simulink model "EcoSIM3_P2_C2_WIP"  (R2014b)
settings: Solver=ode1  SolverMode=SingleTasking  StartTime=0.0  StopTime=4  FixedStep=0.01  RelTol=1e-3
PostLoadFcn:
  | %, if any(exist('dsrtsu_mdlpostloadfcn', 'file') == [2, 3, 6]), try dsrtsu_mdlpostloadfcn('Execute', bdroot); catch fprintf('Error in PostLoadFcn (dsrtsu_mdlpostloadfcn) for model "%s":\n %s\n', bdroot, lasterr); end, end,
InitFcn:
  | tic
  | %Startup_EcoSIM
undefined symbols (not defined in the file or in its folder): canChannel, Controls, DriveCycles, Driver, EM_EFF_MAP, EM_PwrLoss_MAP, EngPwr, EngSpd, EngTrq, Glbl, Overwritten_Mode, Plants, Power, sigbuilder_block, Torque, Trialmap, Veh_Dynamics
libraries: simulink x135, canmsglib x113, fl_lib x104, canlib x89, nesl_utility x56, sdl_lib x29, dspsigops x6, dspswit3 x5, dspstat3 x2, commnoisgen2 x1, dspfdesign x1
(part 11 of 21)

== system EcoSIM3_P2_C2_WIP/Powertrain/Soft_ECUs_IO/From_Goto/Subsystem1/Engine_Relay ==
  In1 : Inport
  Constant4 : Constant
  Constant5 : Constant  Value=0
  Relay2 : Switch  Criteria=u2 > Threshold  Threshold=0.5
  Out1 : Outport
  wires:
  Relay2/1 -> Out1/1  "ICE_Powerup"
  Constant5/1 -> Relay2/3
  Constant4/1 -> Relay2/1
  In1/1 -> Relay2/2

== system EcoSIM3_P2_C2_WIP/Powertrain/Soft_ECUs_IO/VNT Kvaser/CANRx/BAS Receive ==
  Bus Creator12 : BusCreator  Inputs=1
  Bus Creator2 : BusCreator  Inputs=2
  CAN Receive : canlib/CAN Receive  BlockHandle=2745.0026  DeviceMenu=Kvaser Virtual 1 (Channel 1)  Device=Kvaser Virtual 1 (Channel 1)  ObjConstructor=canChannel('Kvaser', 'Virtual 1', 1)  EnableStandardIDsFilter=off  StandardIDs=102  EnableExtendedIDsFilter=off  ExtendedIDs=0  SampleTime=0.01  MsgsPerTimestep=1  StdIDsCombo=Allow only  ExtIDsCombo=Block all  InternalFilterUpdateStatus=on
  CAN Unpack : canmsglib/CAN Unpack  CANdbFile=C:\Users\EcoCAR_HIL\Documents\Khanna\EcoSIM3_P1_0_PHEV_TCU\Final_DBC\Engine_Transmission_BAS.dbc  MsgList=ECO_BAS_Receive_MSG102  MsgName=ECO_BAS_Receive_MSG102  MsgIDType=Standard (11-bit identifier)  MsgIdentifier=102  MsgLength=2  SignalInfo=BAS_Mode_Request$8$1$2$2$1$0$1$0$0$1$#BAS_Torque_Request_Nm$9$15$2$1$1$0$1.000000e-02$0$-1.638400e+02$1.638300e+02$#  NSignals=2  IDPort=off  TimestampPort=off  ErrorPort=off  RemotePort=off  LengthPort=off  StatusPort=off  StartBits=str2num('[int32(8);int32(9)]')  SignalSizes=str2num('[int32(1);int32(15)]')  ByteOrders=str2num('[int32(2);int32(2)]')  DataTypes=str2num('[int32(2);int32(1)]')  MultiplexTypes=str2num('[int32(1);int32(1)]')  MultiplexValues=str2num('[double(0);double(0)]')  Factors=str2num('[double(1);double(1.000000e-02)]')  Offsets=str2num('[double(0);double(0)]')  Minimums=str2num('[double(0);double(-1.638400e+02)]')  Maximums=str2num('[double(1);double(1.638300e+02)]')
      settings: DataFormat=CANdb specified signals
  Terminator6 : Terminator
  BAS_CAN : Outport
  wires:
  Bus Creator12/1 -> BAS_CAN/1  "BAS_CAN"
  Bus Creator2/1 -> Bus Creator12/1  "SetValues"
  CAN Receive/1 -> Terminator6/1
  CAN Unpack/1 -> Bus Creator2/1  "BAS_Mode_Request"
  CAN Unpack/2 -> Bus Creator2/2  "BAS_Torque_Request_Nm"
  CAN Receive/2 -> CAN Unpack/1

== system EcoSIM3_P2_C2_WIP/Powertrain/Soft_ECUs_IO/VNT Kvaser/CANRx/Brusa Receive ==
  Bus Creator4 : BusCreator  Inputs=2
  Ground : Ground
  Ground1 : Ground
  Brusa CAN : Outport
  wires:
  Bus Creator4/1 -> Brusa CAN/1  "Brusa_CAN"
  Ground/1 -> Bus Creator4/1  "Dummy1"
  Ground1/1 -> Bus Creator4/2  "Dummy2"

== system EcoSIM3_P2_C2_WIP/Powertrain/Soft_ECUs_IO/VNT Kvaser/CANRx/EM Receive ==
  Bus Creator : BusCreator  Inputs=1
  Bus Creator1 : BusCreator  Inputs=3
  CAN Receive1 : canlib/CAN Receive  BlockHandle=2767.0024  DeviceMenu=Kvaser Virtual 1 (Channel 2)  Device=Kvaser Virtual 1 (Channel 2)  ObjConstructor=canChannel('Kvaser', 'Virtual 1', 2)  EnableStandardIDsFilter=off  StandardIDs=192  EnableExtendedIDsFilter=off  ExtendedIDs=0  SampleTime=0.01  MsgsPerTimestep=1  StdIDsCombo=Allow only  ExtIDsCombo=Block all  InternalFilterUpdateStatus=on
  CAN Unpack2 : canmsglib/CAN Unpack  CANdbFile=C:\Users\EcoCAR_HIL\Documents\Khanna\EcoSIM3_P1_0_PHEV_TCU\Final_DBC\20150828 RMS PM CAN DB.dbc  MsgList=M192_Command_Message  MsgName=M192_Command_Message  MsgIDType=Standard (11-bit identifier)  MsgIdentifier=192  MsgLength=8  SignalInfo=Direction_Command$42$1$1$2$1$0$1$0$0$1$#Inverter_Discharge$41$1$1$2$1$0$1$0$0$1$#Inverter_Enable$40$1$1$2$1$0$1$0$0$1$#Speed_Command$16$16$1$1$1$0$1$0$-32768$32767$#Torque_Command$0$16$1$1$1$0$1.000000e-01$0$-3.276800e+03$3.276700e+03$#Torque_Limit_Command$48$16$1$1$1$0$1$0$-3.276800e+03$3.276700e+03$#  NSignals=6  IDPort=off  TimestampPort=off  ErrorPort=off  RemotePort=off  LengthPort=off  StatusPort=off  StartBits=str2num('[int32(42);int32(41);int32(40);int32(16);int32(0);int32(48)]')  SignalSizes=str2num('[int32(1);int32(1);int32(1);int32(16);int32(16);int32(16)]')  ByteOrders=str2num('[int32(1);int32(1);int32(1);int32(1);int32(1);int32(1)]')  DataTypes=str2num('[int32(2);int32(2);int32(2);int32(1);int32(1);int32(1)]')  MultiplexTypes=str2num('[int32(1);int32(1);int32(1);int32(1);int32(1);int32(1)]')  MultiplexValues=str2num('[double(0);double(0);double(0);double(0);double(0);double(0)]')  Factors=str2num('[double(1);double(1);double(1);double(1);double(1.000000e-01);double(1)]')  Offsets=str2num('[double(0);double(0);double(0);double(0);double(0);double(0)]')  Minimums=str2num('[double(0);double(0);double(0);double(-32768);double(-3.276800e+03);double(-3.276800e+03)]')  Maximums=str2num('[double(1);double(1);double(1);double(32767);double(3.276700e+03);double(3.276700e+03)]')
      settings: DataFormat=CANdb specified signals
  Terminator{5,7..9} (4 alike) : Terminator
  EM CAN : Outport
  wires:
  Bus Creator/1 -> EM CAN/1  "EM_CAN"
  Bus Creator1/1 -> Bus Creator/1  "M192_Command_Message"
  CAN Receive1/2 -> CAN Unpack2/1
  CAN Receive1/1 -> Terminator5/1
  CAN Unpack2/1 -> Bus Creator1/1  "Rotation_Direction"
  CAN Unpack2/3 -> Bus Creator1/2  "Inverter_Enable"
  CAN Unpack2/5 -> Bus Creator1/3  "Torque_Command"
  CAN Unpack2/2 -> Terminator7/1
  CAN Unpack2/4 -> Terminator8/1
  CAN Unpack2/6 -> Terminator9/1

== system EcoSIM3_P2_C2_WIP/Powertrain/Soft_ECUs_IO/VNT Kvaser/CANRx/ESS Receive ==
  Bus Creator5 : BusCreator
  Bus Creator6 : BusCreator  Inputs=1
  CAN Receive4 : canlib/CAN Receive  BlockHandle=2787.0027  DeviceMenu=Kvaser Virtual 1 (Channel 1)  Device=Kvaser Virtual 1 (Channel 1)  ObjConstructor=canChannel('Kvaser', 'Virtual 1', 1)  EnableStandardIDsFilter=off  StandardIDs=1024  EnableExtendedIDsFilter=off  ExtendedIDs=0  SampleTime=0.01  MsgsPerTimestep=1  StdIDsCombo=Allow only  ExtIDsCombo=Block all  InternalFilterUpdateStatus=on
  CAN Unpack4 : canmsglib/CAN Unpack  CANdbFile=C:\Users\EcoCAR_HIL\Documents\Khanna\EcoSIM3_P1_0_PHEV_TCU\Final_DBC\BCM_VehBus_Std.dbc  MsgList=BCM_Request  MsgName=BCM_Request  MsgIDType=Standard (11-bit identifier)  MsgIdentifier=1024  MsgLength=4  SignalInfo=hsc_bcm_enable$0$1$2$2$1$0$1$0$0$1$#hsc_bcm_epo$1$1$2$2$1$0$1$0$0$1$#hsc_bcm_leakage_ena$3$1$2$2$1$0$1$0$0$1$#hsc_bcm_mainc_close$2$1$2$2$1$0$1$0$0$1$#  NSignals=4  IDPort=off  TimestampPort=off  ErrorPort=off  RemotePort=off  LengthPort=off  StatusPort=off  StartBits=str2num('[int32(0);int32(1);int32(3);int32(2)]')  SignalSizes=str2num('[int32(1);int32(1);int32(1);int32(1)]')  ByteOrders=str2num('[int32(2);int32(2);int32(2);int32(2)]')  DataTypes=str2num('[int32(2);int32(2);int32(2);int32(2)]')  MultiplexTypes=str2num('[int32(1);int32(1);int32(1);int32(1)]')  MultiplexValues=str2num('[double(0);double(0);double(0);double(0)]')  Factors=str2num('[double(1);double(1);double(1);double(1)]')  Offsets=str2num('[double(0);double(0);double(0);double(0)]')  Minimums=str2num('[double(0);double(0);double(0);double(0)]')  Maximums=str2num('[double(1);double(1);double(1);double(1)]')
      settings: DataFormat=CANdb specified signals
  Terminator3 : Terminator
  ESS CAN : Outport
  wires:
  Bus Creator5/1 -> Bus Creator6/1  "BCM_Request"
  Bus Creator6/1 -> ESS CAN/1  "BCM_CAN"
  CAN Receive4/2 -> CAN Unpack4/1
  CAN Receive4/1 -> Terminator3/1
  CAN Unpack4/1 -> Bus Creator5/1  "hsc_bcm_enable"
  CAN Unpack4/2 -> Bus Creator5/2  "hsc_bcm_epo"
  CAN Unpack4/4 -> Bus Creator5/4  "hsc_bcm_mainc_close"
  CAN Unpack4/3 -> Bus Creator5/3  "hsc_bcm_leakage_ena"

== system EcoSIM3_P2_C2_WIP/Powertrain/Soft_ECUs_IO/VNT Kvaser/CANRx/ICE Receive ==
  Bus Creator14 : BusCreator  Inputs=1
  Bus Creator15 : BusCreator  Inputs=1
  CAN Receive2 : canlib/CAN Receive  BlockHandle=2802.0027  DeviceMenu=Kvaser Virtual 1 (Channel 1)  Device=Kvaser Virtual 1 (Channel 1)  ObjConstructor=canChannel('Kvaser', 'Virtual 1', 1)  EnableStandardIDsFilter=off  StandardIDs=101  EnableExtendedIDsFilter=off  ExtendedIDs=0  SampleTime=0.01  MsgsPerTimestep=1  StdIDsCombo=Allow only  ExtIDsCombo=Block all  InternalFilterUpdateStatus=on
  CAN Unpack1 : canmsglib/CAN Unpack  CANdbFile=C:\Users\EcoCAR_HIL\Documents\Khanna\EcoSIM3_P1_0_PHEV_TCU\Final_DBC\Engine_Transmission_BAS.dbc  MsgList=ECO_Engine_MSG101  MsgName=ECO_Engine_MSG101  MsgIDType=Standard (11-bit identifier)  MsgIdentifier=101  MsgLength=2  SignalInfo=ICE_Torque_Request_Nm$9$15$2$2$1$0$1.000000e-02$0$0$3.276700e+02$#  NSignals=1  IDPort=off  TimestampPort=off  ErrorPort=off  RemotePort=off  LengthPort=off  StatusPort=off  StartBits=str2num('[int32(9)]')  SignalSizes=str2num('[int32(15)]')  ByteOrders=str2num('[int32(2)]')  DataTypes=str2num('[int32(2)]')  MultiplexTypes=str2num('[int32(1)]')  MultiplexValues=str2num('[double(0)]')  Factors=str2num('[double(1.000000e-02)]')  Offsets=str2num('[double(0)]')  Minimums=str2num('[double(0)]')  Maximums=str2num('[double(3.276700e+02)]')
      settings: DataFormat=CANdb specified signals
  Terminator11 : Terminator
  ICE CAN : Outport
  wires:
  Bus Creator15/1 -> ICE CAN/1  "ICE_CAN"
  Bus Creator14/1 -> Bus Creator15/1  "ICE_Request"
  CAN Unpack1/1 -> Bus Creator14/1  "ICE_Torque_Request_Nm"
  CAN Receive2/2 -> CAN Unpack1/1
  CAN Receive2/1 -> Terminator11/1

== system EcoSIM3_P2_C2_WIP/Powertrain/Soft_ECUs_IO/VNT Kvaser/CANRx/Transmisssion Receive ==
  Bus Creator : BusCreator  Inputs=2
  Bus Creator18 : BusCreator  Inputs=1
  Bus Creator2 : BusCreator  Inputs=1
  CAN Receive1 : canlib/CAN Receive  BlockHandle=2815.0027  DeviceMenu=Kvaser Virtual 1 (Channel 1)  Device=Kvaser Virtual 1 (Channel 1)  ObjConstructor=canChannel('Kvaser', 'Virtual 1', 1)  EnableStandardIDsFilter=off  StandardIDs=94  EnableExtendedIDsFilter=off  ExtendedIDs=0  SampleTime=0.01  MsgsPerTimestep=1  StdIDsCombo=Allow only  ExtIDsCombo=Block all  InternalFilterUpdateStatus=on
  CAN Receive3 : canlib/CAN Receive  BlockHandle=2816.0023  DeviceMenu=Kvaser Virtual 1 (Channel 1)  Device=Kvaser Virtual 1 (Channel 1)  ObjConstructor=canChannel('Kvaser', 'Virtual 1', 1)  EnableStandardIDsFilter=off  StandardIDs=105  EnableExtendedIDsFilter=off  ExtendedIDs=0  SampleTime=0.01  MsgsPerTimestep=1  StdIDsCombo=Allow only  ExtIDsCombo=Block all  InternalFilterUpdateStatus=on
  CAN Unpack3 : canmsglib/CAN Unpack  CANdbFile=C:\Users\EcoCAR_HIL\Documents\Khanna\EcoSIM3_P1_0_PHEV_TCU\Final_DBC\Engine_Transmission_BAS.dbc  MsgList=ECO_Trans_Receive_MSG105  MsgName=ECO_Trans_Receive_MSG105  MsgIDType=Standard (11-bit identifier)  MsgIdentifier=105  MsgLength=1  SignalInfo=Clutch_Request$4$1$2$2$1$0$1$0$0$1$#Gear_Request$5$3$2$2$1$0$1$0$0$7$#  NSignals=2  IDPort=off  TimestampPort=off  ErrorPort=off  RemotePort=off  LengthPort=off  StatusPort=off  StartBits=str2num('[int32(4);int32(5)]')  SignalSizes=str2num('[int32(1);int32(3)]')  ByteOrders=str2num('[int32(2);int32(2)]')  DataTypes=str2num('[int32(2);int32(2)]')  MultiplexTypes=str2num('[int32(1);int32(1)]')  MultiplexValues=str2num('[double(0);double(0)]')  Factors=str2num('[double(1);double(1)]')  Offsets=str2num('[double(0);double(0)]')  Minimums=str2num('[double(0);double(0)]')  Maximums=str2num('[double(1);double(7)]')
      settings: DataFormat=CANdb specified signals
  CAN Unpack5 : canmsglib/CAN Unpack  CANdbFile=C:\Users\EcoCAR_HIL\Documents\Khanna\EcoSIM3_P1_0_PHEV_TCU\Final_DBC\EcoCAR3_Controls_Development.dbc  MsgList=MABx_Transmit_MSG094  MsgName=MABx_Transmit_MSG094  MsgIDType=Standard (11-bit identifier)  MsgIdentifier=94  MsgLength=1  SignalInfo=Mode$7$1$2$2$1$0$1$0$0$1$#  NSignals=1  IDPort=off  TimestampPort=off  ErrorPort=off  RemotePort=off  LengthPort=off  StatusPort=off  StartBits=str2num('[int32(7)]')  SignalSizes=str2num('[int32(1)]')  ByteOrders=str2num('[int32(2)]')  DataTypes=str2num('[int32(2)]')  MultiplexTypes=str2num('[int32(1)]')  MultiplexValues=str2num('[double(0)]')  Factors=str2num('[double(1)]')  Offsets=str2num('[double(0)]')  Minimums=str2num('[double(0)]')  Maximums=str2num('[double(1)]')
      settings: DataFormat=CANdb specified signals
  Ground : Ground
  Terminator1 : Terminator
  Terminator12 : Terminator
  Terminator13 : Terminator
  Clutch_Trans : Outport
  Mode : Outport  Port=2
  wires:
  Bus Creator18/1 -> Clutch_Trans/1  "Clutch_Trans_CAN"
  Bus Creator/1 -> Mode/1  "Supervisory"
  CAN Unpack5/1 -> Bus Creator/1  "Mode"
  Ground/1 -> Bus Creator/2  "Driver Torque Request"
  CAN Receive3/1 -> Terminator12/1
  Bus Creator2/1 -> Bus Creator18/1  "Trans_Receive"
  CAN Receive3/2 -> CAN Unpack3/1
  CAN Unpack3/2 -> Bus Creator2/1  "Gear_Request"
  CAN Unpack3/1 -> Terminator13/1  "Clutch_Request"
  CAN Receive1/1 -> Terminator1/1
  CAN Receive1/2 -> CAN Unpack5/1

== system EcoSIM3_P2_C2_WIP/Powertrain/Soft_ECUs_IO/VNT Kvaser/CANTx/BAS ==
  BAS : Inport
  Bus Selector5 : BusSelector  OutputSignals=Status_1.BAS_Speed_rad_per_s,Status_1.BAS_Torque_Out_Nm,Status_2.Fault_U,Status_2.Fault_V,Status_2.Fault_W
  CAN Pack5 : canmsglib/CAN Pack  CANdbFile=C:\Users\EcoCAR_HIL\Documents\Khanna\EcoSIM3_P1_0_PHEV_TCU\Final_DBC\Engine_Transmission_BAS.dbc  MsgList=ECO_BAS_Status_MSG099  MsgName=ECO_BAS_Status_MSG099  MsgIDType=Standard (11-bit identifier)  MsgIdentifier=99  MsgLength=5  SignalInfo=BAS_Fault_Status$36$1$2$2$1$0$1$0$0$1$#BAS_Speed_rad_per_s$8$16$2$1$1$0$1.000000e-01$0$-3.276800e+03$3.276700e+03$#BAS_Status_Mode$37$1$2$2$1$0$1$0$0$1$#BAS_Torque_Command_Nm$25$15$2$1$1$0$1.000000e-02$0$-1.638400e+02$1.638300e+02$#Fault_U$24$1$2$2$1$0$1$0$0$1$#Fault_V$39$1$2$2$1$0$1$0$0$1$#Fault_W$38$1$2$2$1$0$1$0$0$1$#  NSignals=7  StartBits=str2num('[int32(36);int32(8);int32(37);int32(25);int32(24);int32(39);int32(38)]')  SignalSizes=str2num('[int32(1);int32(16);int32(1);int32(15);int32(1);int32(1);int32(1)]')  ByteOrders=str2num('[int32(2);int32(2);int32(2);int32(2);int32(2);int32(2);int32(2)]')  DataTypes=str2num('[int32(2);int32(1);int32(2);int32(1);int32(2);int32(2);int32(2)]')  MultiplexTypes=str2num('[int32(1);int32(1);int32(1);int32(1);int32(1);int32(1);int32(1)]')  MultiplexValues=str2num('[double(0);double(0);double(0);double(0);double(0);double(0);double(0)]')  Factors=str2num('[double(1);double(1.000000e-01);double(1);double(1.000000e-02);double(1);double(1);double(1)]')  Offsets=str2num('[double(0);double(0);double(0);double(0);double(0);double(0);double(0)]')  Minimums=str2num('[double(0);double(-3.276800e+03);double(0);double(-1.638400e+02);double(0);double(0);double(0)]')  Maximums=str2num('[double(1);double(3.276700e+03);double(1);double(1.638300e+02);double(1);double(1);double(1)]')  Remote=off
      settings: DataFormat=CANdb specified signals
  CAN Transmit5 : canlib/CAN Transmit  BlockHandle=2851.0023  DeviceMenu=Kvaser Virtual 1 (Channel 1)  Device=Kvaser Virtual 1 (Channel 1)  ObjConstructor=canChannel('Kvaser', 'Virtual 1', 1)  EnablePeriodicTransmit=off  MessagePeriod=1.000
  Ground_1 : Ground
  Ground_2 : Ground
  wires:
  Ground_2/1 -> CAN Pack5/3
  Ground_1/1 -> CAN Pack5/1
  Bus Selector5/5 -> CAN Pack5/7  "<Fault_W>"
  Bus Selector5/4 -> CAN Pack5/6  "<Fault_V>"
  Bus Selector5/3 -> CAN Pack5/5  "<Fault_U>"
  Bus Selector5/2 -> CAN Pack5/4  "<BAS_Torque_Out_Nm>"
  Bus Selector5/1 -> CAN Pack5/2  "<BAS_Speed_rad_per_s>"
  BAS/1 -> Bus Selector5/1
  CAN Pack5/1 -> CAN Transmit5/1

== system EcoSIM3_P2_C2_WIP/Powertrain/Soft_ECUs_IO/VNT Kvaser/CANTx/Brusa ==
  Brusa : Inport
  Bus Selector5 : BusSelector  OutputSignals=Brusa_Dummy_msg.Dummy1,Brusa_Dummy_msg.Dummy2
  Terminator : Terminator
  Terminator1 : Terminator
  wires:
  Brusa/1 -> Bus Selector5/1
  Bus Selector5/1 -> Terminator/1  "<Dummy1>"
  Bus Selector5/2 -> Terminator1/1  "<Dummy2>"

== system EcoSIM3_P2_C2_WIP/Powertrain/Soft_ECUs_IO/VNT Kvaser/CANTx/Clutch_and_Trans ==
  Trans : Inport
  Bus Selector4 : BusSelector  OutputSignals=Message_1.Actual_Gear
  CAN Pack3 : canmsglib/CAN Pack  CANdbFile=C:\Users\EcoCAR_HIL\Documents\Khanna\EcoSIM3_P1_0_PHEV_TCU\Final_DBC\Engine_Transmission_BAS.dbc  MsgList=ECO_Trans_Status_MSG106  MsgName=ECO_Trans_Status_MSG106  MsgIDType=Standard (11-bit identifier)  MsgIdentifier=106  MsgLength=1  SignalInfo=Actual_Gear$1$3$2$2$1$0$1$0$0$7$#Clutch_Sw$7$1$2$2$1$0$1$0$0$1$#TCM_Gear$4$3$2$2$1$0$1$0$0$7$#  NSignals=3  StartBits=str2num('[int32(1);int32(7);int32(4)]')  SignalSizes=str2num('[int32(3);int32(1);int32(3)]')  ByteOrders=str2num('[int32(2);int32(2);int32(2)]')  DataTypes=str2num('[int32(2);int32(2);int32(2)]')  MultiplexTypes=str2num('[int32(1);int32(1);int32(1)]')  MultiplexValues=str2num('[double(0);double(0);double(0)]')  Factors=str2num('[double(1);double(1);double(1)]')  Offsets=str2num('[double(0);double(0);double(0)]')  Minimums=str2num('[double(0);double(0);double(0)]')  Maximums=str2num('[double(7);double(1);double(7)]')  Remote=off
      settings: DataFormat=CANdb specified signals
  CAN Transmit3 : canlib/CAN Transmit  BlockHandle=2876.0023  DeviceMenu=Kvaser Virtual 1 (Channel 1)  Device=Kvaser Virtual 1 (Channel 1)  ObjConstructor=canChannel('Kvaser', 'Virtual 1', 1)  EnablePeriodicTransmit=off  MessagePeriod=1.000
  Ground10 : Ground
  Ground11 : Ground
  wires:
  Ground11/1 -> CAN Pack3/3
  Ground10/1 -> CAN Pack3/2
  Bus Selector4/1 -> CAN Pack3/1  "<Actual_Gear>"
  CAN Pack3/1 -> CAN Transmit3/1
  Trans/1 -> Bus Selector4/1

== system EcoSIM3_P2_C2_WIP/Powertrain/Soft_ECUs_IO/VNT Kvaser/CANTx/EM ==
  EM : Inport
  M160_Temperature_Set_1 : Subsystem
  M161_Temperature_Set_2 : Subsystem
  M162_Temperature_Set_3 : Subsystem
  M165_Motor_Position_Info : Subsystem
  M170_Internal_States : Subsystem
  M171_Fault_Codes : Subsystem
  M172_Torque_And_Timer_Info : Subsystem
  wires:
  EM/1 -> M160_Temperature_Set_1/1(EM), M161_Temperature_Set_2/1(EM), M162_Temperature_Set_3/1(EM), M170_Internal_States/1(EM), M172_Torque_And_Timer_Info/1(EM), M165_Motor_Position_Info/1(EM), M171_Fault_Codes/1(EM)

== system EcoSIM3_P2_C2_WIP/Powertrain/Soft_ECUs_IO/VNT Kvaser/CANTx/ESS ==
  ESS : Inport
  BCM_Data : Subsystem
  BCM_Limits : Subsystem
  BCM_Status : Subsystem
  wires:
  ESS/1 -> BCM_Data/1(ESS), BCM_Status/1(ESS), BCM_Limits/1(ESS)

== system EcoSIM3_P2_C2_WIP/Powertrain/Soft_ECUs_IO/VNT Kvaser/CANTx/Engine ==
  ICE : Inport
  Bus Selector1 : BusSelector  OutputSignals=ICE_Torque.ICE_Torque_Cmd_Nm
  CAN Pack : canmsglib/CAN Pack  CANdbFile=C:\Users\EcoCAR_HIL\Documents\Khanna\EcoSIM3_P1_0_PHEV_TCU\Final_DBC\Engine_Transmission_BAS.dbc  MsgList=ECO_Engine_MSG104  MsgName=ECO_Engine_MSG104  MsgIDType=Standard (11-bit identifier)  MsgIdentifier=104  MsgLength=2  SignalInfo=ICE_Torque_Cmd_Nm$9$15$2$2$1$0$1.000000e-02$0$0$3.276700e+02$#  NSignals=1  StartBits=str2num('[int32(9)]')  SignalSizes=str2num('[int32(15)]')  ByteOrders=str2num('[int32(2)]')  DataTypes=str2num('[int32(2)]')  MultiplexTypes=str2num('[int32(1)]')  MultiplexValues=str2num('[double(0)]')  Factors=str2num('[double(1.000000e-02)]')  Offsets=str2num('[double(0)]')  Minimums=str2num('[double(0)]')  Maximums=str2num('[double(3.276700e+02)]')  Remote=off
      settings: DataFormat=CANdb specified signals
  CAN Transmit : canlib/CAN Transmit  BlockHandle=3132.0018  DeviceMenu=Kvaser Virtual 1 (Channel 1)  Device=Kvaser Virtual 1 (Channel 1)  ObjConstructor=canChannel('Kvaser', 'Virtual 1', 1)  EnablePeriodicTransmit=off  MessagePeriod=1.000
  wires:
  CAN Pack/1 -> CAN Transmit/1
  Bus Selector1/1 -> CAN Pack/1  "<ICE_Torque_Cmd_Nm>"
  ICE/1 -> Bus Selector1/1

== system EcoSIM3_P2_C2_WIP/Powertrain/Soft_ECUs_IO/VNT Kvaser/CANTx/GMLAN ==
  Driver : Inport
  PPEI_Brake_Apply_Status : Subsystem
  PPEI_Driven_Whl_Rotational_Stat : Subsystem
  PPEI_NonDrivn_Whl_Rotationl_Stat : Subsystem
  PPEI_Platform_General_Status : Subsystem
  PPEI_Vehicle_Speed_and_Distance : Subsystem
  wires:
  Driver/1 -> PPEI_Vehicle_Speed_and_Distance/1(GM), PPEI_NonDrivn_Whl_Rotationl_Stat/1(GM), PPEI_Driven_Whl_Rotational_Stat/1(GM), PPEI_Platform_General_Status/1(GM), PPEI_Brake_Apply_Status/1(GM)

== system EcoSIM3_P2_C2_WIP/Powertrain/Soft_ECUs_IO/VNT Kvaser/ElectricalRx/BAS_Relay ==
  In1 : Inport
  Constant6 : Constant
  Constant7 : Constant  Value=0
  Relay3 : Switch  Criteria=u2 > Threshold  Threshold=0.5
  Out1 : Outport
  wires:
  In1/1 -> Relay3/2
  Constant7/1 -> Relay3/3
  Relay3/1 -> Out1/1  "BAS_Powerup"
  Constant6/1 -> Relay3/1

== system EcoSIM3_P2_C2_WIP/Powertrain/Soft_ECUs_IO/VNT Kvaser/ElectricalRx/EM_Relay ==
  In1 : Inport
  Constant2 : Constant
  Constant3 : Constant  Value=0
  Relay1 : Switch  Criteria=u2 > Threshold  Threshold=0.5
  Out1 : Outport
  wires:
  In1/1 -> Relay1/2
  Constant3/1 -> Relay1/3
  Constant2/1 -> Relay1/1
  Relay1/1 -> Out1/1  "EM_Powerup"

== system EcoSIM3_P2_C2_WIP/Powertrain/Soft_ECUs_IO/VNT Kvaser/ElectricalRx/Engine_Relay ==
  In1 : Inport
  Constant4 : Constant
  Constant5 : Constant  Value=0
  Relay2 : Switch  Criteria=u2 > Threshold  Threshold=0.5
  Out1 : Outport
  wires:
  In1/1 -> Relay2/2
  Constant4/1 -> Relay2/1
  Constant5/1 -> Relay2/3
  Relay2/1 -> Out1/1  "ICE_Powerup"

== system EcoSIM3_P2_C2_WIP/Powertrain/Soft_ECUs_IO/VNT Vector/CANRx/BAS Receive ==
  Bus Creator1 : BusCreator  Inputs=2
  Bus Creator12 : BusCreator  Inputs=2
  Bus Creator2 : BusCreator  Inputs=3
  CAN Receive : canlib/CAN Receive  BlockHandle=11427.0005  DeviceMenu=Vector Virtual 1 (Channel 1)  Device=Vector Virtual 1 (Channel 1)  ObjConstructor=canChannel('Vector', 'Virtual 1', 1)  EnableStandardIDsFilter=off  StandardIDs=[256 272]  EnableExtendedIDsFilter=off  ExtendedIDs=0  SampleTime=0.01  MsgsPerTimestep=all  StdIDsCombo=Allow only  ExtIDsCombo=Block all  InternalFilterUpdateStatus=on
  CAN Unpack : canmsglib/CAN Unpack  CANdbFile=C:\Box Sync\EcoCAR 3\SMS\EcoSIM3_P2_C2\MIL\Final_DBC\InfineonInverter.dbc  MsgList=SetValues  MsgName=SetValues  MsgIDType=Standard (11-bit identifier)  MsgIdentifier=256  MsgLength=8  SignalInfo=Checksum1$0$8$1$2$1$0$1$0$-Inf$Inf$#Counter1$8$8$1$2$1$0$1$0$0$15$#ID_Command$32$16$1$1$3$1$3.125000e-02$0$-1024$1.023969e+03$#IQ_Command$16$16$1$1$3$1$3.125000e-02$0$-1024$1.023969e+03$#ModeReq$48$8$1$2$2$0$1$0$0$2$#Reserved1$56$8$1$2$1$0$1$0$0$255$#Speed_Command$16$16$1$1$3$2$5.000000e-01$0$-16384$1.638350e+04$#  NSignals=7  IDPort=off  TimestampPort=off  ErrorPort=off  RemotePort=off  LengthPort=off  StatusPort=off  StartBits=str2num('[int32(0);int32(8);int32(32);int32(16);int32(48);int32(56);int32(16)]')  SignalSizes=str2num('[int32(8);int32(8);int32(16);int32(16);int32(8);int32(8);int32(16)]')  ByteOrders=str2num('[int32(1);int32(1);int32(1);int32(1);int32(1);int32(1);int32(1)]')  DataTypes=str2num('[int32(2);int32(2);int32(1);int32(1);int32(2);int32(2);int32(1)]')  MultiplexTypes=str2num('[int32(1);int32(1);int32(3);int32(3);int32(2);int32(1);int32(3)]')  MultiplexValues=str2num('[double(0);double(0);double(1);double(1);double(0);double(0);double(2)]')  Factors=str2num('[double(1);double(1);double(3.125000e-02);double(3.125000e-02);double(1);double(1);double(5.000000e-01)]')  Offsets=str2num('[double(0);double(0);double(0);double(0);double(0);double(0);double(0)]')  Minimums=str2num('[double(-Inf);double(0);double(-1024);double(-1024);double(0);double(0);double(-16384)]')  Maximums=str2num('[double(Inf);double(15);double(1.023969e+03);double(1.023969e+03);double(2);double(255);double(1.638350e+04)]')
      settings: DataFormat=CANdb specified signals
  CAN Unpack1 : canmsglib/CAN Unpack  CANdbFile=C:\Box Sync\EcoCAR 3\SMS\EcoSIM3_P2_C2\MIL\Final_DBC\InfineonInverter.dbc  MsgList=SetLimits  MsgName=SetLimits  MsgIDType=Standard (11-bit identifier)  MsgIdentifier=272  MsgLength=8  SignalInfo=Checksum2$0$8$1$2$1$0$1$0$0$255$#Code$16$8$1$2$2$0$1$0$0$2$#Counter2$8$4$1$2$1$0$1$0$0$15$#ID_Limit$48$16$1$1$3$1$3.125000e-02$0$-1024$1.023969e+03$#IQ_Limit$32$16$1$1$3$1$3.125000e-02$0$-1024$1.023969e+03$#Reserved2$12$2$1$2$1$0$1$0$0$3$#Reserved3$15$1$1$2$1$0$1$0$0$1$#Write$14$1$1$2$1$0$1$0$0$1$#  NSignals=8  IDPort=off  TimestampPort=off  ErrorPort=off  RemotePort=off  LengthPort=off  StatusPort=off  StartBits=str2num('[int32(0);int32(16);int32(8);int32(48);int32(32);int32(12);int32(15);int32(14)]')  SignalSizes=str2num('[int32(8);int32(8);int32(4);int32(16);int32(16);int32(2);int32(1);int32(1)]')  ByteOrders=str2num('[int32(1);int32(1);int32(1);int32(1);int32(1);int32(1);int32(1);int32(1)]')  DataTypes=str2num('[int32(2);int32(2);int32(2);int32(1);int32(1);int32(2);int32(2);int32(2)]')  MultiplexTypes=str2num('[int32(1);int32(2);int32(1);int32(3);int32(3);int32(1);int32(1);int32(1)]')  MultiplexValues=str2num('[double(0);double(0);double(0);double(1);double(1);double(0);double(0);double(0)]')  Factors=str2num('[double(1);double(1);double(1);double(3.125000e-02);double(3.125000e-02);double(1);double(1);double(1)]')  Offsets=str2num('[double(0);double(0);double(0);double(0);double(0);double(0);double(0);double(0)]')  Minimums=str2num('[double(0);double(0);double(0);double(-1024);double(-1024);double(0);double(0);double(0)]')  Maximums=str2num('[double(255);double(2);double(15);double(1.023969e+03);double(1.023969e+03);double(3);double(1);double(1)]')
      settings: DataFormat=CANdb specified signals
  Terminator6 : Terminator
  Terminator_{2..11} (10 alike) : Terminator
  BAS_CAN : Outport
  wires:
  Bus Creator12/1 -> BAS_CAN/1  "BAS_CAN"
  Bus Creator2/1 -> Bus Creator12/1  "SetValues"
  CAN Receive/1 -> Terminator6/1
  CAN Receive/2 -> CAN Unpack1/1, CAN Unpack/1
  CAN Unpack/3 -> Bus Creator2/1  "ID_Command"
  CAN Unpack/4 -> Bus Creator2/2  "IQ_Command"
  CAN Unpack/5 -> Bus Creator2/3  "ModeReq"
  CAN Unpack1/4 -> Bus Creator1/1  "ID_Limit"
  CAN Unpack1/5 -> Bus Creator1/2  "IQ_Limit"
  Bus Creator1/1 -> Bus Creator12/2  "SetLimits"
  CAN Unpack/1 -> Terminator_2/1  "BAS_Mode_Request"
  CAN Unpack/2 -> Terminator_3/1  "BAS_Torque_Request_Nm"
  CAN Unpack/6 -> Terminator_4/1
  CAN Unpack/7 -> Terminator_5/1
  CAN Unpack1/1 -> Terminator_6/1
  CAN Unpack1/2 -> Terminator_7/1
  CAN Unpack1/3 -> Terminator_8/1
  CAN Unpack1/6 -> Terminator_9/1
  CAN Unpack1/7 -> Terminator_10/1
  CAN Unpack1/8 -> Terminator_11/1

== system EcoSIM3_P2_C2_WIP/Powertrain/Soft_ECUs_IO/VNT Vector/CANRx/Brusa Receive ==
  Bus Creator4 : BusCreator  Inputs=2
  Ground : Ground
  Ground1 : Ground
  Brusa CAN : Outport
  wires:
  Bus Creator4/1 -> Brusa CAN/1  "Brusa_CAN"
  Ground/1 -> Bus Creator4/1  "Dummy1"
  Ground1/1 -> Bus Creator4/2  "Dummy2"

== system EcoSIM3_P2_C2_WIP/Powertrain/Soft_ECUs_IO/VNT Vector/CANRx/EM Receive ==
  Bus Creator : BusCreator  Inputs=1
  Bus Creator1 : BusCreator  Inputs=3
  CAN Receive1 : canlib/CAN Receive  BlockHandle=11476.0005  DeviceMenu=Vector Virtual 1 (Channel 2)  Device=Vector Virtual 1 (Channel 2)  ObjConstructor=canChannel('Vector', 'Virtual 1', 2)  EnableStandardIDsFilter=off  StandardIDs=192  EnableExtendedIDsFilter=off  ExtendedIDs=0  SampleTime=0.01  MsgsPerTimestep=1  StdIDsCombo=Allow only  ExtIDsCombo=Block all  InternalFilterUpdateStatus=on
  CAN Unpack2 : canmsglib/CAN Unpack  CANdbFile=C:\Users\EcoCAR_HIL\Documents\Khanna\EcoSIM3_P1_0_PHEV_TCU\Final_DBC\20160113 RMS PM CAN DB.dbc  MsgList=M192_Command_Message  MsgName=M192_Command_Message  MsgIDType=Standard (11-bit identifier)  MsgIdentifier=192  MsgLength=8  SignalInfo=Direction_Command$32$1$1$2$1$0$1$0$0$1$#Inverter_Discharge$41$1$1$2$1$0$1$0$0$1$#Inverter_Enable$40$1$1$2$1$0$1$0$0$1$#Speed_Command$16$16$1$1$1$0$1$0$-32768$32767$#Speed_Mode_Enable$42$1$1$2$1$0$1$0$0$1$#Torque_Command$0$16$1$1$1$0$1.000000e-01$0$-3.276800e+03$3.276700e+03$#Torque_Limit_Command$48$16$1$1$1$0$1$0$-3.276800e+03$3.276700e+03$#  NSignals=7  IDPort=off  TimestampPort=off  ErrorPort=off  RemotePort=off  LengthPort=off  StatusPort=off  StartBits=str2num('[int32(32);int32(41);int32(40);int32(16);int32(42);int32(0);int32(48)]')  SignalSizes=str2num('[int32(1);int32(1);int32(1);int32(16);int32(1);int32(16);int32(16)]')  ByteOrders=str2num('[int32(1);int32(1);int32(1);int32(1);int32(1);int32(1);int32(1)]')  DataTypes=str2num('[int32(2);int32(2);int32(2);int32(1);int32(2);int32(1);int32(1)]')  MultiplexTypes=str2num('[int32(1);int32(1);int32(1);int32(1);int32(1);int32(1);int32(1)]')  MultiplexValues=str2num('[double(0);double(0);double(0);double(0);double(0);double(0);double(0)]')  Factors=str2num('[double(1);double(1);double(1);double(1);double(1);double(1.000000e-01);double(1)]')  Offsets=str2num('[double(0);double(0);double(0);double(0);double(0);double(0);double(0)]')  Minimums=str2num('[double(0);double(0);double(0);double(-32768);double(0);double(-3.276800e+03);double(-3.276800e+03)]')  Maximums=str2num('[double(1);double(1);double(1);double(32767);double(1);double(3.276700e+03);double(3.276700e+03)]')
      settings: DataFormat=CANdb specified signals
  Terminator5 : Terminator
  Terminator_{2..5} (4 alike) : Terminator
  EM CAN : Outport
  wires:
  Bus Creator/1 -> EM CAN/1  "EM_CAN"
  Bus Creator1/1 -> Bus Creator/1  "M192_Command_Message"
  CAN Receive1/2 -> CAN Unpack2/1
  CAN Receive1/1 -> Terminator5/1
  CAN Unpack2/1 -> Bus Creator1/1  "Rotation_Direction"
  CAN Unpack2/3 -> Bus Creator1/2  "Inverter_Enable"
  CAN Unpack2/6 -> Bus Creator1/3  "Torque_Command"
  CAN Unpack2/2 -> Terminator_2/1
  CAN Unpack2/4 -> Terminator_3/1
  CAN Unpack2/5 -> Terminator_4/1
  CAN Unpack2/7 -> Terminator_5/1

== system EcoSIM3_P2_C2_WIP/Powertrain/Soft_ECUs_IO/VNT Vector/CANRx/ESS-DCDC Receive ==
  Bus Creator1 : BusCreator  Inputs=3
  Bus Creator2 : BusCreator  Inputs=1
  Bus Creator5 : BusCreator
  Bus Creator6 : BusCreator  Inputs=1
  CAN Receive4 : canlib/CAN Receive  BlockHandle=6974.0007  DeviceMenu=Vector Virtual 1 (Channel 1)  Device=Vector Virtual 1 (Channel 1)  ObjConstructor=canChannel('Vector', 'Virtual 1', 1)  EnableStandardIDsFilter=off  StandardIDs=[1024 468]  EnableExtendedIDsFilter=off  ExtendedIDs=0  SampleTime=0.01  MsgsPerTimestep=all  StdIDsCombo=Allow only  ExtIDsCombo=Block all  InternalFilterUpdateStatus=on
  CAN Unpack1 : canmsglib/CAN Unpack  CANdbFile=C:\Box Sync\EcoCAR 3\SMS\EcoSIM3_P2_C2\MIL\Final_DBC\GlobalA_v4p3_APM_PE_v2.dbc  MsgList=PTEI_Hybrid_General_Status_1  MsgName=PTEI_Hybrid_General_Status_1  MsgIDType=Standard (11-bit identifier)  MsgIdentifier=468  MsgLength=2  SignalInfo=HybContClrLgsDiag$6$1$2$2$1$0$1$0$0$1$#LowVoltEnblRq$7$1$2$2$1$0$1$0$0$1$#LwVltStpntCmnd$8$8$2$2$1$0$7.843140e-02$0$0$2.000001e+01$#PrplsnSysAtv$5$1$2$2$1$0$1$0$0$1$#  NSignals=4  IDPort=off  TimestampPort=off  ErrorPort=off  RemotePort=off  LengthPort=off  StatusPort=off  StartBits=str2num('[int32(6);int32(7);int32(8);int32(5)]')  SignalSizes=str2num('[int32(1);int32(1);int32(8);int32(1)]')  ByteOrders=str2num('[int32(2);int32(2);int32(2);int32(2)]')  DataTypes=str2num('[int32(2);int32(2);int32(2);int32(2)]')  MultiplexTypes=str2num('[int32(1);int32(1);int32(1);int32(1)]')  MultiplexValues=str2num('[double(0);double(0);double(0);double(0)]')  Factors=str2num('[double(1);double(1);double(7.843140e-02);double(1)]')  Offsets=str2num('[double(0);double(0);double(0);double(0)]')  Minimums=str2num('[double(0);double(0);double(0);double(0)]')  Maximums=str2num('[double(1);double(1);double(2.000001e+01);double(1)]')
      settings: DataFormat=CANdb specified signals
  CAN Unpack4 : canmsglib/CAN Unpack  CANdbFile=C:\Users\EcoCAR_HIL\Documents\Khanna\EcoSIM3_P1_0_PHEV_TCU\Final_DBC\BCM_VehBus_Std.dbc  MsgList=BCM_Request  MsgName=BCM_Request  MsgIDType=Standard (11-bit identifier)  MsgIdentifier=1024  MsgLength=4  SignalInfo=hsc_bcm_enable$0$1$2$2$1$0$1$0$0$1$#hsc_bcm_epo$1$1$2$2$1$0$1$0$0$1$#hsc_bcm_leakage_ena$3$1$2$2$1$0$1$0$0$1$#hsc_bcm_mainc_close$2$1$2$2$1$0$1$0$0$1$#  NSignals=4  IDPort=off  TimestampPort=off  ErrorPort=off  RemotePort=off  LengthPort=off  StatusPort=off  StartBits=str2num('[int32(0);int32(1);int32(3);int32(2)]')  SignalSizes=str2num('[int32(1);int32(1);int32(1);int32(1)]')  ByteOrders=str2num('[int32(2);int32(2);int32(2);int32(2)]')  DataTypes=str2num('[int32(2);int32(2);int32(2);int32(2)]')  MultiplexTypes=str2num('[int32(1);int32(1);int32(1);int32(1)]')  MultiplexValues=str2num('[double(0);double(0);double(0);double(0)]')  Factors=str2num('[double(1);double(1);double(1);double(1)]')  Offsets=str2num('[double(0);double(0);double(0);double(0)]')  Minimums=str2num('[double(0);double(0);double(0);double(0)]')  Maximums=str2num('[double(1);double(1);double(1);double(1)]')
      settings: DataFormat=CANdb specified signals
  Terminator : Terminator
  Terminator3 : Terminator
  ESS CAN : Outport
  DCDC CAN : Outport  Port=2
  wires:
  Bus Creator5/1 -> Bus Creator6/1  "BCM_Request"
  Bus Creator6/1 -> ESS CAN/1  "BCM_CAN"
  CAN Receive4/2 -> CAN Unpack1/1, CAN Unpack4/1
  CAN Receive4/1 -> Terminator3/1
  CAN Unpack4/1 -> Bus Creator5/1  "hsc_bcm_enable"
  CAN Unpack4/2 -> Bus Creator5/2  "hsc_bcm_epo"
  CAN Unpack4/4 -> Bus Creator5/4  "hsc_bcm_mainc_close"
  CAN Unpack4/3 -> Bus Creator5/3  "hsc_bcm_leakage_ena"
  CAN Unpack1/4 -> Bus Creator1/3  "PrplsnSysAtv"
  CAN Unpack1/3 -> Bus Creator1/2  "LwVltStpntCmnd"
  CAN Unpack1/2 -> Bus Creator1/1  "LowVoltEnblRq"
  CAN Unpack1/1 -> Terminator/1
  Bus Creator1/1 -> Bus Creator2/1  "PTEI_Hybrid_General_Status_1"
  Bus Creator2/1 -> DCDC CAN/1  "DCDC_CAN"

== system EcoSIM3_P2_C2_WIP/Powertrain/Soft_ECUs_IO/VNT Vector/CANRx/ICE Receive ==
  Bus Creator14 : BusCreator  Inputs=3
  Bus Creator15 : BusCreator  Inputs=1
  CAN Receive2 : canlib/CAN Receive  BlockHandle=11526.0007  DeviceMenu=Vector Virtual 1 (Channel 1)  Device=Vector Virtual 1 (Channel 1)  ObjConstructor=canChannel('Vector', 'Virtual 1', 1)  EnableStandardIDsFilter=off  StandardIDs=101  EnableExtendedIDsFilter=off  ExtendedIDs=0  SampleTime=0.01  MsgsPerTimestep=1  StdIDsCombo=Allow only  ExtIDsCombo=Block all  InternalFilterUpdateStatus=on
  CAN Unpack1 : canmsglib/CAN Unpack  CANdbFile=C:\Users\EcoCAR_HIL\Documents\Khanna\EcoSIM3_P1_0_PHEV_TCU\Final_DBC\Engine_Transmission_BAS.dbc  MsgList=ECO_Engine_MSG101  MsgName=ECO_Engine_MSG101  MsgIDType=Standard (11-bit identifier)  MsgIdentifier=101  MsgLength=3  SignalInfo=ICE_Torque_Request_Nm$9$15$2$2$1$0$1.000000e-02$0$0$3.276700e+02$#ISP_R$8$1$2$2$1$0$1$0$0$1$#PCM_Wake$23$1$2$2$1$0$1$0$0$1$#  NSignals=3  IDPort=off  TimestampPort=off  ErrorPort=off  RemotePort=off  LengthPort=off  StatusPort=off  StartBits=str2num('[int32(9);int32(8);int32(23)]')  SignalSizes=str2num('[int32(15);int32(1);int32(1)]')  ByteOrders=str2num('[int32(2);int32(2);int32(2)]')  DataTypes=str2num('[int32(2);int32(2);int32(2)]')  MultiplexTypes=str2num('[int32(1);int32(1);int32(1)]')  MultiplexValues=str2num('[double(0);double(0);double(0)]')  Factors=str2num('[double(1.000000e-02);double(1);double(1)]')  Offsets=str2num('[double(0);double(0);double(0)]')  Minimums=str2num('[double(0);double(0);double(0)]')  Maximums=str2num('[double(3.276700e+02);double(1);double(1)]')
      settings: DataFormat=CANdb specified signals
  Gain : Gain
  Gain1 : Gain
  Terminator11 : Terminator
  ICE CAN : Outport
  wires:
  Bus Creator15/1 -> ICE CAN/1  "ICE_CAN"
  Bus Creator14/1 -> Bus Creator15/1  "ICE_Request"
  CAN Unpack1/1 -> Bus Creator14/1  "ICE_Torque_Request_Nm"
  CAN Receive2/2 -> CAN Unpack1/1
  CAN Receive2/1 -> Terminator11/1
  Gain/1 -> Bus Creator14/2  "ISP_R"
  Gain1/1 -> Bus Creator14/3  "PCM_Wake"
  CAN Unpack1/2 -> Gain/1
  CAN Unpack1/3 -> Gain1/1

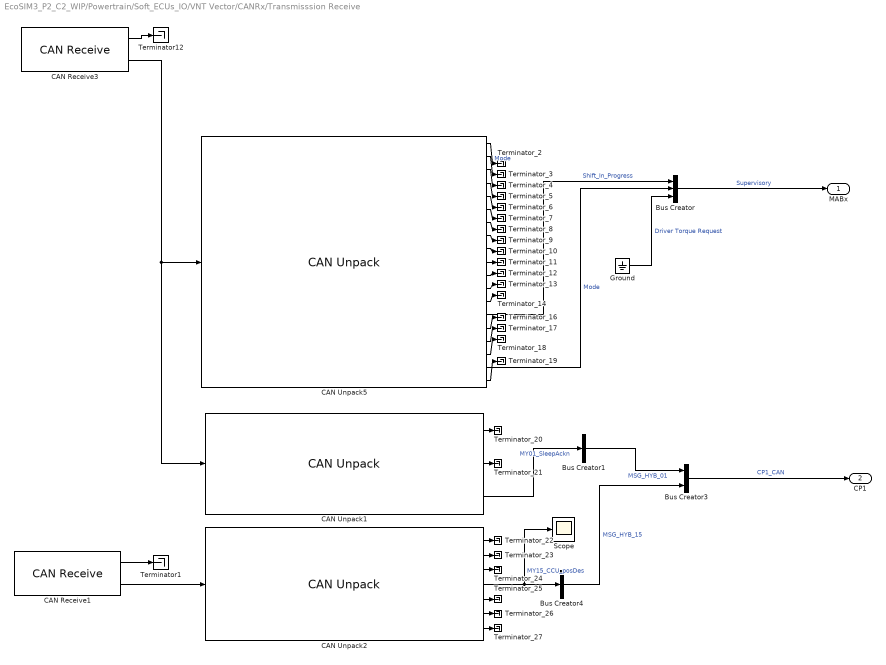
== system EcoSIM3_P2_C2_WIP/Powertrain/Soft_ECUs_IO/VNT Vector/CANRx/Transmisssion Receive ==
  Bus Creator : BusCreator  Inputs=3
  Bus Creator1 : BusCreator  Inputs=1
  Bus Creator3 : BusCreator  Inputs=2
  Bus Creator4 : BusCreator  Inputs=1
  CAN Receive1 : canlib/CAN Receive  BlockHandle=11546.0007  DeviceMenu=Vector Virtual 1 (Channel 1)  Device=Vector Virtual 1 (Channel 1)  ObjConstructor=canChannel('Vector', 'Virtual 1', 1)  EnableStandardIDsFilter=off  StandardIDs=150  EnableExtendedIDsFilter=off  ExtendedIDs=0  SampleTime=0.01  MsgsPerTimestep=all  StdIDsCombo=Allow only  ExtIDsCombo=Block all  InternalFilterUpdateStatus=on
  CAN Receive3 : canlib/CAN Receive  BlockHandle=11547.0004  DeviceMenu=Vector Virtual 1 (Channel 1)  Device=Vector Virtual 1 (Channel 1)  ObjConstructor=canChannel('Vector', 'Virtual 1', 1)  EnableStandardIDsFilter=off  StandardIDs=[94 105 150 934]  EnableExtendedIDsFilter=off  ExtendedIDs=0  SampleTime=0.01  MsgsPerTimestep=all  StdIDsCombo=Allow only  ExtIDsCombo=Block all  InternalFilterUpdateStatus=on
  CAN Unpack1 : canmsglib/CAN Unpack  CANdbFile=C:\Box Sync\EcoCAR 3\SMS\EcoSIM3_P2_C2\MIL\Final_DBC\FTE_ElecHydAct.dbc  MsgList=MSG_HYB_01  MsgName=MSG_HYB_01  MsgIDType=Standard (11-bit identifier)  MsgIdentifier=934  MsgLength=8  SignalInfo=MY01_Checksum$0$8$1$2$1$0$1$0$-Inf$Inf$#MY01_Counter$8$4$1$2$1$0$1$0$0$15$#MY01_SleepAckn$12$1$1$2$1$0$1$0$-Inf$Inf$#  NSignals=3  IDPort=off  TimestampPort=off  ErrorPort=off  RemotePort=off  LengthPort=off  StatusPort=off  StartBits=str2num('[int32(0);int32(8);int32(12)]')  SignalSizes=str2num('[int32(8);int32(4);int32(1)]')  ByteOrders=str2num('[int32(1);int32(1);int32(1)]')  DataTypes=str2num('[int32(2);int32(2);int32(2)]')  MultiplexTypes=str2num('[int32(1);int32(1);int32(1)]')  MultiplexValues=str2num('[double(0);double(0);double(0)]')  Factors=str2num('[double(1);double(1);double(1)]')  Offsets=str2num('[double(0);double(0);double(0)]')  Minimums=str2num('[double(-Inf);double(0);double(-Inf)]')  Maximums=str2num('[double(Inf);double(15);double(Inf)]')
      settings: DataFormat=CANdb specified signals
  CAN Unpack2 : canmsglib/CAN Unpack  CANdbFile=C:\Box Sync\EcoCAR 3\SMS\EcoSIM3_P2_C2\MIL\Final_DBC\FTE_ElecHydAct.dbc  MsgList=MSG_HYB_15  MsgName=MSG_HYB_15  MsgIDType=Standard (11-bit identifier)  MsgIdentifier=150  MsgLength=8  SignalInfo=MY15_CCU_pLimReq$15$1$1$2$1$0$1$0$-Inf$Inf$#MY15_CCU_pMax$20$4$1$2$1$0$1$0$-Inf$Inf$#MY15_CCU_pMin$16$4$1$2$1$0$1$0$-Inf$Inf$#MY15_CCU_posDes$24$13$1$2$1$0$1$0$0$6327$#MY15_CCU_stModeReq$12$3$1$2$1$0$1$0$-Inf$Inf$#MY15_Checksum$0$8$1$2$1$0$1$0$-Inf$Inf$#MY15_Counter$8$4$1$2$1$0$1$0$-Inf$Inf$#  NSignals=7  IDPort=off  TimestampPort=off  ErrorPort=off  RemotePort=off  LengthPort=off  StatusPort=off  StartBits=str2num('[int32(15);int32(20);int32(16);int32(24);int32(12);int32(0);int32(8)]')  SignalSizes=str2num('[int32(1);int32(4);int32(4);int32(13);int32(3);int32(8);int32(4)]')  ByteOrders=str2num('[int32(1);int32(1);int32(1);int32(1);int32(1);int32(1);int32(1)]')  DataTypes=str2num('[int32(2);int32(2);int32(2);int32(2);int32(2);int32(2);int32(2)]')  MultiplexTypes=str2num('[int32(1);int32(1);int32(1);int32(1);int32(1);int32(1);int32(1)]')  MultiplexValues=str2num('[double(0);double(0);double(0);double(0);double(0);double(0);double(0)]')  Factors=str2num('[double(1);double(1);double(1);double(1);double(1);double(1);double(1)]')  Offsets=str2num('[double(0);double(0);double(0);double(0);double(0);double(0);double(0)]')  Minimums=str2num('[double(-Inf);double(-Inf);double(-Inf);double(0);double(-Inf);double(-Inf);double(-Inf)]')  Maximums=str2num('[double(Inf);double(Inf);double(Inf);double(6327);double(Inf);double(Inf);double(Inf)]')
      settings: DataFormat=CANdb specified signals
  CAN Unpack5 : canmsglib/CAN Unpack  CANdbFile=C:\Box Sync\EcoCAR 3\SMS\EcoSIM3_P2_C2\MIL\Final_DBC\EcoCAR3_Controls_Development.dbc  MsgList=MABx_Transmit_MSG094  MsgName=MABx_Transmit_MSG094  MsgIDType=Standard (11-bit identifier)  MsgIdentifier=94  MsgLength=4  SignalInfo=Charge_Sustain_Switch$23$1$2$2$1$0$1$0$0$1$#Charging_Complete$11$1$2$2$1$0$1$0$0$1$#Charging_Light$10$1$2$2$1$0$1$0$0$1$#EPB_Disengage_Pulse$16$1$2$2$1$0$1$0$0$1$#EPB_Engage_Pulse$17$1$2$2$1$0$1$0$0$1$#Eng_Fuel_Pump$19$1$2$2$1$0$1$0$0$1$#Eng_Fusebox$18$1$2$2$1$0$1$0$0$1$#Engine_On_Switch$22$1$2$2$1$0$1$0$0$1$#GFD_Light$9$1$2$2$1$0$1$0$0$1$#MABx_Heartbeat$2$5$2$2$1$0$1$0$0$31$#Mode$7$1$2$2$1$0$1$0$0$1$#PRNDL$29$3$2$2$1$0$1$0$0$5$#Regen_Disable_Switch$21$1$2$2$1$0$1$0$0$1$#Shift_In_Progress$28$1$2$2$1$0$1$0$0$1$#Shutdown_Complete$20$1$2$2$1$0$1$0$0$1$#Starter_Request$0$1$2$2$1$0$1$0$0$1$#Veh_Relay_Request$1$1$2$2$1$0$1$0$0$1$#Vehicle_Mode$12$4$2$2$1$0$1$0$0$15$#Vehicle_Ready_Light$8$1$2$2$1$0$1$0$0$1$#  NSignals=19  IDPort=off  TimestampPort=off  ErrorPort=off  RemotePort=off  LengthPort=off  StatusPort=off  StartBits=str2num('[int32(23);int32(11);int32(10);int32(16);int32(17);int32(19);int32(18);int32(22);int32(9);int32(2);int32(7);int32(29);int32(21);int32(28);int32(20);int32(0);int32(1);int32(12);int32(8)]')  SignalSizes=str2num('[int32(1);int32(1);int32(1);int32(1);int32(1);int32(1);int32(1);int32(1);int32(1);int32(5);int32(1);int32(3);int32(1);int32(1);int32(1);int32(1);int32(1);int32(4);int32(1)]')  ByteOrders=str2num('[int32(2);int32(2);int32(2);int32(2);int32(2);int32(2);int32(2);int32(2);int32(2);int32(2);int32(2);int32(2);int32(2);int32(2);int32(2);int32(2);int32(2);int32(2);int32(2)]')  DataTypes=str2num('[int32(2);int32(2);int32(2);int32(2);int32(2);int32(2);int32(2);int32(2);int32(2);int32(2);int32(2);int32(2);int32(2);int32(2);int32(2);int32(2);int32(2);int32(2);int32(2)]')  MultiplexTypes=str2num('[int32(1);int32(1);int32(1);int32(1);int32(1);int32(1);int32(1);int32(1);int32(1);int32(1);int32(1);int32(1);int32(1);int32(1);int32(1);int32(1);int32(1);int32(1);int32(1)]')  MultiplexValues=str2num('[double(0);double(0);double(0);double(0);double(0);double(0);double(0);double(0);double(0);double(0);double(0);double(0);double(0);double(0);double(0);double(0);double(0);double(0);double(0)]')  Factors=str2num('[double(1);double(1);double(1);double(1);double(1);double(1);double(1);double(1);double(1);double(1);double(1);double(1);double(1);double(1);double(1);double(1);double(1);double(1);double(1)]')  Offsets=str2num('[double(0);double(0);double(0);double(0);double(0);double(0);double(0);double(0);double(0);double(0);double(0);double(0);double(0);double(0);double(0);double(0);double(0);double(0);double(0)]')  Minimums=str2num('[double(0);double(0);double(0);double(0);double(0);double(0);double(0);double(0);double(0);double(0);double(0);double(0);double(0);double(0);double(0);double(0);double(0);double(0);double(0)]')  Maximums=str2num('[double(1);double(1);double(1);double(1);double(1);double(1);double(1);double(1);double(1);double(31);double(1);double(5);double(1);double(1);double(1);double(1);double(1);double(15);double(1)]')
      settings: DataFormat=CANdb specified signals
  Ground : Ground
  Scope : Scope
      settings: SaveName=ScopeData53
  Terminator1 : Terminator
  Terminator12 : Terminator
  Terminator_{2..14,16..27} (25 alike) : Terminator
  MABx : Outport
  CP1 : Outport  Port=2
  wires:
  Bus Creator/1 -> MABx/1  "Supervisory"
  CAN Unpack5/18 -> Bus Creator/2  "Mode"
  Ground/1 -> Bus Creator/3  "Driver Torque Request"
  CAN Receive3/1 -> Terminator12/1
  CAN Unpack5/1 -> Terminator_2/1  "Mode"
  CAN Unpack5/2 -> Terminator_3/1
  CAN Unpack5/3 -> Terminator_4/1
  CAN Unpack5/4 -> Terminator_5/1
  CAN Unpack5/5 -> Terminator_6/1
  CAN Unpack5/6 -> Terminator_7/1
  CAN Unpack5/7 -> Terminator_8/1
  CAN Unpack5/8 -> Terminator_9/1
  CAN Unpack5/9 -> Terminator_10/1
  CAN Unpack5/10 -> Terminator_11/1
  CAN Unpack5/11 -> Terminator_12/1
  CAN Unpack5/12 -> Terminator_13/1
  CAN Unpack5/13 -> Terminator_14/1
  CAN Unpack5/15 -> Terminator_16/1
  CAN Unpack5/16 -> Terminator_17/1
  CAN Unpack5/17 -> Terminator_18/1
  CAN Unpack5/19 -> Terminator_19/1
  CAN Unpack5/14 -> Bus Creator/1  "Shift_In_Progress"
  CAN Receive3/2 -> CAN Unpack1/1, CAN Unpack5/1
  CAN Unpack1/3 -> Bus Creator1/1  "MY01_SleepAckn"
  CAN Unpack2/4 -> Scope/1, Bus Creator4/1  "MY15_CCU_posDes"
  Bus Creator1/1 -> Bus Creator3/1  "MSG_HYB_01"
  Bus Creator4/1 -> Bus Creator3/2  "MSG_HYB_15"
  Bus Creator3/1 -> CP1/1  "CP1_CAN"
  CAN Unpack1/1 -> Terminator_20/1
  CAN Unpack1/2 -> Terminator_21/1
  CAN Unpack2/1 -> Terminator_22/1
  CAN Unpack2/2 -> Terminator_23/1
  CAN Unpack2/3 -> Terminator_24/1
  CAN Unpack2/5 -> Terminator_25/1
  CAN Unpack2/6 -> Terminator_26/1
  CAN Unpack2/7 -> Terminator_27/1
  CAN Receive1/2 -> CAN Unpack2/1
  CAN Receive1/1 -> Terminator1/1

== system EcoSIM3_P2_C2_WIP/Powertrain/Soft_ECUs_IO/VNT Vector/CANTx/BAS ==
  BAS : Inport
  CAN Transmit5 : canlib/CAN Transmit  BlockHandle=11638.0004  DeviceMenu=Vector Virtual 1 (Channel 1)  Device=Vector Virtual 1 (Channel 1)  ObjConstructor=canChannel('Vector', 'Virtual 1', 1)  EnablePeriodicTransmit=off  MessagePeriod=1.000
  Mux : Mux  Inputs=2
  Status_1 : Subsystem
  Status_2 : Subsystem
  wires:
  BAS/1 -> Status_2/1(In1), Status_1/1(In1)
  Status_1/1(Out1) -> Mux/1
  Status_2/1(Out1) -> Mux/2
  Mux/1 -> CAN Transmit5/1

== system EcoSIM3_P2_C2_WIP/Powertrain/Soft_ECUs_IO/VNT Vector/CANTx/Brusa ==
  Brusa : Inport
  Bus Selector5 : BusSelector  OutputSignals=Brusa_Dummy_msg.Dummy1,Brusa_Dummy_msg.Dummy2
  Terminator : Terminator
  Terminator1 : Terminator
  wires:
  Brusa/1 -> Bus Selector5/1
  Bus Selector5/1 -> Terminator/1  "<Dummy1>"
  Bus Selector5/2 -> Terminator1/1  "<Dummy2>"

== system EcoSIM3_P2_C2_WIP/Powertrain/Soft_ECUs_IO/VNT Vector/CANTx/Clutch_and_Trans ==
  CP1 : Inport
  Bus Selector1 : BusSelector  OutputSignals=CCU_HYB_01.CY01_posCurr,CCU_HYB_01.CY01_stMode
  CAN Pack1 : canmsglib/CAN Pack  CANdbFile=C:\Box Sync\EcoCAR 3\SMS\EcoSIM3_P2_C2\MIL\Final_DBC\FTE_ElecHydAct.dbc  MsgList=CCU_HYB_01  MsgName=CCU_HYB_01  MsgIDType=Standard (11-bit identifier)  MsgIdentifier=127  MsgLength=8  SignalInfo=CY01_AngSpdCurr$24$9$1$2$1$0$200$-51000$-51000$50800$#CY01_Checksum$0$8$1$2$1$0$1$0$-Inf$Inf$#CY01_Counter$8$4$1$2$1$0$1$0$0$15$#CY01_ErrCAN$35$1$1$2$1$0$1$0$-Inf$Inf$#CY01_ErrHW$33$1$1$2$1$0$1$0$-Inf$Inf$#CY01_ErrMech$34$1$1$2$1$0$1$0$-Inf$Inf$#CY01_ErrTempHigh$38$1$1$2$1$0$1$0$-Inf$Inf$#CY01_ErrTempWarn$37$1$1$2$1$0$1$0$-Inf$Inf$#CY01_ErrUBattLow$36$1$1$2$1$0$1$0$-Inf$Inf$#CY01_SleepInd$39$1$1$2$1$0$1$0$-Inf$Inf$#CY01_i2trqCurr$12$12$1$2$1$0$2.500000e-01$-511$-511$5.122500e+02$#CY01_pCurr$56$8$1$2$1$0$2.000000e-01$0$0$5.060000e+01$#CY01_posCurr$40$13$1$2$1$0$1$0$0$8191$#CY01_stMode$53$3$1$2$1$0$1$0$0$7$#  NSignals=14  StartBits=str2num('[int32(24);int32(0);int32(8);int32(35);int32(33);int32(34);int32(38);int32(37);int32(36);int32(39);int32(12);int32(56);int32(40);int32(53)]')  SignalSizes=str2num('[int32(9);int32(8);int32(4);int32(1);int32(1);int32(1);int32(1);int32(1);int32(1);int32(1);int32(12);int32(8);int32(13);int32(3)]')  ByteOrders=str2num('[int32(1);int32(1);int32(1);int32(1);int32(1);int32(1);int32(1);int32(1);int32(1);int32(1);int32(1);int32(1);int32(1);int32(1)]')  DataTypes=str2num('[int32(2);int32(2);int32(2);int32(2);int32(2);int32(2);int32(2);int32(2);int32(2);int32(2);int32(2);int32(2);int32(2);int32(2)]')  MultiplexTypes=str2num('[int32(1);int32(1);int32(1);int32(1);int32(1);int32(1);int32(1);int32(1);int32(1);int32(1);int32(1);int32(1);int32(1);int32(1)]')  MultiplexValues=str2num('[double(0);double(0);double(0);double(0);double(0);double(0);double(0);double(0);double(0);double(0);double(0);double(0);double(0);double(0)]')  Factors=str2num('[double(200);double(1);double(1);double(1);double(1);double(1);double(1);double(1);double(1);double(1);double(2.500000e-01);double(2.000000e-01);double(1);double(1)]')  Offsets=str2num('[double(-51000);double(0);double(0);double(0);double(0);double(0);double(0);double(0);double(0);double(0);double(-511);double(0);double(0);double(0)]')  Minimums=str2num('[double(-51000);double(-Inf);double(0);double(-Inf);double(-Inf);double(-Inf);double(-Inf);double(-Inf);double(-Inf);double(-Inf);double(-511);double(0);double(0);double(0)]')  Maximums=str2num('[double(50800);double(Inf);double(15);double(Inf);double(Inf);double(Inf);double(Inf);double(Inf);double(Inf);double(Inf);double(5.122500e+02);double(5.060000e+01);double(8191);double(7)]')  Remote=off
      settings: DataFormat=CANdb specified signals
  CAN Transmit3 : canlib/CAN Transmit  BlockHandle=11740.0004  DeviceMenu=Vector Virtual 1 (Channel 1)  Device=Vector Virtual 1 (Channel 1)  ObjConstructor=canChannel('Vector', 'Virtual 1', 1)  EnablePeriodicTransmit=off  MessagePeriod=1.000
  Rate Transition : RateTransition
  Rate Transition1 : RateTransition
  wires:
  CP1/1 -> Bus Selector1/1
  Bus Selector1/2 -> Rate Transition/1  "<CY01_stMode>"
  Rate Transition/1 -> CAN Pack1/14
  Bus Selector1/1 -> Rate Transition1/1  "<CY01_posCurr>"
  Rate Transition1/1 -> CAN Pack1/13
  CAN Pack1/1 -> CAN Transmit3/1
